simulink model "c960x4096_x14_7_r2013b_frb"  (R2013b)
settings: Solver=ode45  StartTime=0.0  StopTime=40960  RelTol=1e-3
undefined symbols (not defined in the file): sfp
libraries: xbsIndex_r4 x14620, casper_library_misc x61, dspsigops x32, casper_library_multipliers x24, simulink x18, xps_library x18
(part 70 of 79)

== system c960x4096_x14_7_r2013b_frb/vacc/vacc/yy/bit_sel2/bus_expand1 ==
  bus_in : Inport
  reinterpret{1..64} (64 alike) : xbsIndex_r4/Reinterpret  force_arith_type=on  arith_type=Unsigned  force_bin_pt=on  bin_pt=0  block_type=reinterpret
  slice1 : xbsIndex_r4/Slice  nbits=1  boolean_output=off  mode=Upper Bit Location + Width  bit1=-63  base1=MSB of Input  bit0=0  base0=LSB of Input  dbl_ovrd=off  block_type=slice
  slice10 : xbsIndex_r4/Slice  nbits=1  boolean_output=off  mode=Upper Bit Location + Width  bit1=-54  base1=MSB of Input  bit0=0  base0=LSB of Input  dbl_ovrd=off  block_type=slice
  slice11 : xbsIndex_r4/Slice  nbits=1  boolean_output=off  mode=Upper Bit Location + Width  bit1=-53  base1=MSB of Input  bit0=0  base0=LSB of Input  dbl_ovrd=off  block_type=slice
  slice12 : xbsIndex_r4/Slice  nbits=1  boolean_output=off  mode=Upper Bit Location + Width  bit1=-52  base1=MSB of Input  bit0=0  base0=LSB of Input  dbl_ovrd=off  block_type=slice
  slice13 : xbsIndex_r4/Slice  nbits=1  boolean_output=off  mode=Upper Bit Location + Width  bit1=-51  base1=MSB of Input  bit0=0  base0=LSB of Input  dbl_ovrd=off  block_type=slice
  slice14 : xbsIndex_r4/Slice  nbits=1  boolean_output=off  mode=Upper Bit Location + Width  bit1=-50  base1=MSB of Input  bit0=0  base0=LSB of Input  dbl_ovrd=off  block_type=slice
  slice15 : xbsIndex_r4/Slice  nbits=1  boolean_output=off  mode=Upper Bit Location + Width  bit1=-49  base1=MSB of Input  bit0=0  base0=LSB of Input  dbl_ovrd=off  block_type=slice
  slice16 : xbsIndex_r4/Slice  nbits=1  boolean_output=off  mode=Upper Bit Location + Width  bit1=-48  base1=MSB of Input  bit0=0  base0=LSB of Input  dbl_ovrd=off  block_type=slice
  slice17 : xbsIndex_r4/Slice  nbits=1  boolean_output=off  mode=Upper Bit Location + Width  bit1=-47  base1=MSB of Input  bit0=0  base0=LSB of Input  dbl_ovrd=off  block_type=slice
  slice18 : xbsIndex_r4/Slice  nbits=1  boolean_output=off  mode=Upper Bit Location + Width  bit1=-46  base1=MSB of Input  bit0=0  base0=LSB of Input  dbl_ovrd=off  block_type=slice
  slice19 : xbsIndex_r4/Slice  nbits=1  boolean_output=off  mode=Upper Bit Location + Width  bit1=-45  base1=MSB of Input  bit0=0  base0=LSB of Input  dbl_ovrd=off  block_type=slice
  slice2 : xbsIndex_r4/Slice  nbits=1  boolean_output=off  mode=Upper Bit Location + Width  bit1=-62  base1=MSB of Input  bit0=0  base0=LSB of Input  dbl_ovrd=off  block_type=slice
  slice20 : xbsIndex_r4/Slice  nbits=1  boolean_output=off  mode=Upper Bit Location + Width  bit1=-44  base1=MSB of Input  bit0=0  base0=LSB of Input  dbl_ovrd=off  block_type=slice
  slice21 : xbsIndex_r4/Slice  nbits=1  boolean_output=off  mode=Upper Bit Location + Width  bit1=-43  base1=MSB of Input  bit0=0  base0=LSB of Input  dbl_ovrd=off  block_type=slice
  slice22 : xbsIndex_r4/Slice  nbits=1  boolean_output=off  mode=Upper Bit Location + Width  bit1=-42  base1=MSB of Input  bit0=0  base0=LSB of Input  dbl_ovrd=off  block_type=slice
  slice23 : xbsIndex_r4/Slice  nbits=1  boolean_output=off  mode=Upper Bit Location + Width  bit1=-41  base1=MSB of Input  bit0=0  base0=LSB of Input  dbl_ovrd=off  block_type=slice
  slice24 : xbsIndex_r4/Slice  nbits=1  boolean_output=off  mode=Upper Bit Location + Width  bit1=-40  base1=MSB of Input  bit0=0  base0=LSB of Input  dbl_ovrd=off  block_type=slice
  slice25 : xbsIndex_r4/Slice  nbits=1  boolean_output=off  mode=Upper Bit Location + Width  bit1=-39  base1=MSB of Input  bit0=0  base0=LSB of Input  dbl_ovrd=off  block_type=slice
  slice26 : xbsIndex_r4/Slice  nbits=1  boolean_output=off  mode=Upper Bit Location + Width  bit1=-38  base1=MSB of Input  bit0=0  base0=LSB of Input  dbl_ovrd=off  block_type=slice
  slice27 : xbsIndex_r4/Slice  nbits=1  boolean_output=off  mode=Upper Bit Location + Width  bit1=-37  base1=MSB of Input  bit0=0  base0=LSB of Input  dbl_ovrd=off  block_type=slice
  slice28 : xbsIndex_r4/Slice  nbits=1  boolean_output=off  mode=Upper Bit Location + Width  bit1=-36  base1=MSB of Input  bit0=0  base0=LSB of Input  dbl_ovrd=off  block_type=slice
  slice29 : xbsIndex_r4/Slice  nbits=1  boolean_output=off  mode=Upper Bit Location + Width  bit1=-35  base1=MSB of Input  bit0=0  base0=LSB of Input  dbl_ovrd=off  block_type=slice
  slice3 : xbsIndex_r4/Slice  nbits=1  boolean_output=off  mode=Upper Bit Location + Width  bit1=-61  base1=MSB of Input  bit0=0  base0=LSB of Input  dbl_ovrd=off  block_type=slice
  slice30 : xbsIndex_r4/Slice  nbits=1  boolean_output=off  mode=Upper Bit Location + Width  bit1=-34  base1=MSB of Input  bit0=0  base0=LSB of Input  dbl_ovrd=off  block_type=slice
  slice31 : xbsIndex_r4/Slice  nbits=1  boolean_output=off  mode=Upper Bit Location + Width  bit1=-33  base1=MSB of Input  bit0=0  base0=LSB of Input  dbl_ovrd=off  block_type=slice
  slice32 : xbsIndex_r4/Slice  nbits=1  boolean_output=off  mode=Upper Bit Location + Width  bit1=-32  base1=MSB of Input  bit0=0  base0=LSB of Input  dbl_ovrd=off  block_type=slice
  slice33 : xbsIndex_r4/Slice  nbits=1  boolean_output=off  mode=Upper Bit Location + Width  bit1=-31  base1=MSB of Input  bit0=0  base0=LSB of Input  dbl_ovrd=off  block_type=slice
  slice34 : xbsIndex_r4/Slice  nbits=1  boolean_output=off  mode=Upper Bit Location + Width  bit1=-30  base1=MSB of Input  bit0=0  base0=LSB of Input  dbl_ovrd=off  block_type=slice
  slice35 : xbsIndex_r4/Slice  nbits=1  boolean_output=off  mode=Upper Bit Location + Width  bit1=-29  base1=MSB of Input  bit0=0  base0=LSB of Input  dbl_ovrd=off  block_type=slice
  slice36 : xbsIndex_r4/Slice  nbits=1  boolean_output=off  mode=Upper Bit Location + Width  bit1=-28  base1=MSB of Input  bit0=0  base0=LSB of Input  dbl_ovrd=off  block_type=slice
  slice37 : xbsIndex_r4/Slice  nbits=1  boolean_output=off  mode=Upper Bit Location + Width  bit1=-27  base1=MSB of Input  bit0=0  base0=LSB of Input  dbl_ovrd=off  block_type=slice
  slice38 : xbsIndex_r4/Slice  nbits=1  boolean_output=off  mode=Upper Bit Location + Width  bit1=-26  base1=MSB of Input  bit0=0  base0=LSB of Input  dbl_ovrd=off  block_type=slice
  slice39 : xbsIndex_r4/Slice  nbits=1  boolean_output=off  mode=Upper Bit Location + Width  bit1=-25  base1=MSB of Input  bit0=0  base0=LSB of Input  dbl_ovrd=off  block_type=slice
  slice4 : xbsIndex_r4/Slice  nbits=1  boolean_output=off  mode=Upper Bit Location + Width  bit1=-60  base1=MSB of Input  bit0=0  base0=LSB of Input  dbl_ovrd=off  block_type=slice
  slice40 : xbsIndex_r4/Slice  nbits=1  boolean_output=off  mode=Upper Bit Location + Width  bit1=-24  base1=MSB of Input  bit0=0  base0=LSB of Input  dbl_ovrd=off  block_type=slice
  slice41 : xbsIndex_r4/Slice  nbits=1  boolean_output=off  mode=Upper Bit Location + Width  bit1=-23  base1=MSB of Input  bit0=0  base0=LSB of Input  dbl_ovrd=off  block_type=slice
  slice42 : xbsIndex_r4/Slice  nbits=1  boolean_output=off  mode=Upper Bit Location + Width  bit1=-22  base1=MSB of Input  bit0=0  base0=LSB of Input  dbl_ovrd=off  block_type=slice
  slice43 : xbsIndex_r4/Slice  nbits=1  boolean_output=off  mode=Upper Bit Location + Width  bit1=-21  base1=MSB of Input  bit0=0  base0=LSB of Input  dbl_ovrd=off  block_type=slice
  slice44 : xbsIndex_r4/Slice  nbits=1  boolean_output=off  mode=Upper Bit Location + Width  bit1=-20  base1=MSB of Input  bit0=0  base0=LSB of Input  dbl_ovrd=off  block_type=slice
  slice45 : xbsIndex_r4/Slice  nbits=1  boolean_output=off  mode=Upper Bit Location + Width  bit1=-19  base1=MSB of Input  bit0=0  base0=LSB of Input  dbl_ovrd=off  block_type=slice
  slice46 : xbsIndex_r4/Slice  nbits=1  boolean_output=off  mode=Upper Bit Location + Width  bit1=-18  base1=MSB of Input  bit0=0  base0=LSB of Input  dbl_ovrd=off  block_type=slice
  slice47 : xbsIndex_r4/Slice  nbits=1  boolean_output=off  mode=Upper Bit Location + Width  bit1=-17  base1=MSB of Input  bit0=0  base0=LSB of Input  dbl_ovrd=off  block_type=slice
  slice48 : xbsIndex_r4/Slice  nbits=1  boolean_output=off  mode=Upper Bit Location + Width  bit1=-16  base1=MSB of Input  bit0=0  base0=LSB of Input  dbl_ovrd=off  block_type=slice
  slice49 : xbsIndex_r4/Slice  nbits=1  boolean_output=off  mode=Upper Bit Location + Width  bit1=-15  base1=MSB of Input  bit0=0  base0=LSB of Input  dbl_ovrd=off  block_type=slice
  slice5 : xbsIndex_r4/Slice  nbits=1  boolean_output=off  mode=Upper Bit Location + Width  bit1=-59  base1=MSB of Input  bit0=0  base0=LSB of Input  dbl_ovrd=off  block_type=slice
  slice50 : xbsIndex_r4/Slice  nbits=1  boolean_output=off  mode=Upper Bit Location + Width  bit1=-14  base1=MSB of Input  bit0=0  base0=LSB of Input  dbl_ovrd=off  block_type=slice
  slice51 : xbsIndex_r4/Slice  nbits=1  boolean_output=off  mode=Upper Bit Location + Width  bit1=-13  base1=MSB of Input  bit0=0  base0=LSB of Input  dbl_ovrd=off  block_type=slice
  slice52 : xbsIndex_r4/Slice  nbits=1  boolean_output=off  mode=Upper Bit Location + Width  bit1=-12  base1=MSB of Input  bit0=0  base0=LSB of Input  dbl_ovrd=off  block_type=slice
  slice53 : xbsIndex_r4/Slice  nbits=1  boolean_output=off  mode=Upper Bit Location + Width  bit1=-11  base1=MSB of Input  bit0=0  base0=LSB of Input  dbl_ovrd=off  block_type=slice
  slice54 : xbsIndex_r4/Slice  nbits=1  boolean_output=off  mode=Upper Bit Location + Width  bit1=-10  base1=MSB of Input  bit0=0  base0=LSB of Input  dbl_ovrd=off  block_type=slice
  slice55 : xbsIndex_r4/Slice  nbits=1  boolean_output=off  mode=Upper Bit Location + Width  bit1=-9  base1=MSB of Input  bit0=0  base0=LSB of Input  dbl_ovrd=off  block_type=slice
  slice56 : xbsIndex_r4/Slice  nbits=1  boolean_output=off  mode=Upper Bit Location + Width  bit1=-8  base1=MSB of Input  bit0=0  base0=LSB of Input  dbl_ovrd=off  block_type=slice
  slice57 : xbsIndex_r4/Slice  nbits=1  boolean_output=off  mode=Upper Bit Location + Width  bit1=-7  base1=MSB of Input  bit0=0  base0=LSB of Input  dbl_ovrd=off  block_type=slice
  slice58 : xbsIndex_r4/Slice  nbits=1  boolean_output=off  mode=Upper Bit Location + Width  bit1=-6  base1=MSB of Input  bit0=0  base0=LSB of Input  dbl_ovrd=off  block_type=slice
  slice59 : xbsIndex_r4/Slice  nbits=1  boolean_output=off  mode=Upper Bit Location + Width  bit1=-5  base1=MSB of Input  bit0=0  base0=LSB of Input  dbl_ovrd=off  block_type=slice
  slice6 : xbsIndex_r4/Slice  nbits=1  boolean_output=off  mode=Upper Bit Location + Width  bit1=-58  base1=MSB of Input  bit0=0  base0=LSB of Input  dbl_ovrd=off  block_type=slice
  slice60 : xbsIndex_r4/Slice  nbits=1  boolean_output=off  mode=Upper Bit Location + Width  bit1=-4  base1=MSB of Input  bit0=0  base0=LSB of Input  dbl_ovrd=off  block_type=slice
  slice61 : xbsIndex_r4/Slice  nbits=1  boolean_output=off  mode=Upper Bit Location + Width  bit1=-3  base1=MSB of Input  bit0=0  base0=LSB of Input  dbl_ovrd=off  block_type=slice
  slice62 : xbsIndex_r4/Slice  nbits=1  boolean_output=off  mode=Upper Bit Location + Width  bit1=-2  base1=MSB of Input  bit0=0  base0=LSB of Input  dbl_ovrd=off  block_type=slice
  slice63 : xbsIndex_r4/Slice  nbits=1  boolean_output=off  mode=Upper Bit Location + Width  bit1=-1  base1=MSB of Input  bit0=0  base0=LSB of Input  dbl_ovrd=off  block_type=slice
  slice64 : xbsIndex_r4/Slice  nbits=1  boolean_output=off  mode=Upper Bit Location + Width  bit1=0  base1=MSB of Input  bit0=0  base0=LSB of Input  dbl_ovrd=off  block_type=slice
  slice7 : xbsIndex_r4/Slice  nbits=1  boolean_output=off  mode=Upper Bit Location + Width  bit1=-57  base1=MSB of Input  bit0=0  base0=LSB of Input  dbl_ovrd=off  block_type=slice
  slice8 : xbsIndex_r4/Slice  nbits=1  boolean_output=off  mode=Upper Bit Location + Width  bit1=-56  base1=MSB of Input  bit0=0  base0=LSB of Input  dbl_ovrd=off  block_type=slice
  slice9 : xbsIndex_r4/Slice  nbits=1  boolean_output=off  mode=Upper Bit Location + Width  bit1=-55  base1=MSB of Input  bit0=0  base0=LSB of Input  dbl_ovrd=off  block_type=slice
  msb_out64 : Outport
  out63 : Outport  Port=2
  out62 : Outport  Port=3
  out61 : Outport  Port=4
  out60 : Outport  Port=5
  out59 : Outport  Port=6
  out58 : Outport  Port=7
  out57 : Outport  Port=8
  out56 : Outport  Port=9
  out55 : Outport  Port=10
  out54 : Outport  Port=11
  out53 : Outport  Port=12
  out52 : Outport  Port=13
  out51 : Outport  Port=14
  out50 : Outport  Port=15
  out49 : Outport  Port=16
  out48 : Outport  Port=17
  out47 : Outport  Port=18
  out46 : Outport  Port=19
  out45 : Outport  Port=20
  out44 : Outport  Port=21
  out43 : Outport  Port=22
  out42 : Outport  Port=23
  out41 : Outport  Port=24
  out40 : Outport  Port=25
  out39 : Outport  Port=26
  out38 : Outport  Port=27
  out37 : Outport  Port=28
  out36 : Outport  Port=29
  out35 : Outport  Port=30
  out34 : Outport  Port=31
  out33 : Outport  Port=32
  out32 : Outport  Port=33
  out31 : Outport  Port=34
  out30 : Outport  Port=35
  out29 : Outport  Port=36
  out28 : Outport  Port=37
  out27 : Outport  Port=38
  out26 : Outport  Port=39
  out25 : Outport  Port=40
  out24 : Outport  Port=41
  out23 : Outport  Port=42
  out22 : Outport  Port=43
  out21 : Outport  Port=44
  out20 : Outport  Port=45
  out19 : Outport  Port=46
  out18 : Outport  Port=47
  out17 : Outport  Port=48
  out16 : Outport  Port=49
  out15 : Outport  Port=50
  out14 : Outport  Port=51
  out13 : Outport  Port=52
  out12 : Outport  Port=53
  out11 : Outport  Port=54
  out10 : Outport  Port=55
  out9 : Outport  Port=56
  out8 : Outport  Port=57
  out7 : Outport  Port=58
  out6 : Outport  Port=59
  out5 : Outport  Port=60
  out4 : Outport  Port=61
  out3 : Outport  Port=62
  out2 : Outport  Port=63
  lsb_out1 : Outport  Port=64
  wires:
  bus_in/1 -> slice64/1, slice63/1, slice62/1, slice61/1, slice60/1, slice59/1, slice58/1, slice57/1, slice56/1, slice55/1, slice54/1, slice53/1, slice52/1, slice51/1, slice50/1, slice49/1, slice48/1, slice47/1, slice46/1, slice45/1, slice44/1, slice43/1, slice42/1, slice41/1, slice40/1, slice39/1, slice38/1, slice37/1, slice36/1, slice35/1, slice34/1, slice33/1, slice32/1, slice31/1, slice30/1, slice29/1, slice28/1, slice27/1, slice26/1, slice25/1, slice24/1, slice23/1, slice22/1, slice21/1, slice20/1, slice19/1, slice18/1, slice17/1, slice16/1, slice15/1, slice14/1, slice13/1, slice12/1, slice11/1, slice10/1, slice9/1, slice8/1, slice7/1, slice6/1, slice5/1, slice4/1, slice3/1, slice2/1, slice1/1
  slice64/1 -> reinterpret64/1
  reinterpret64/1 -> msb_out64/1
  slice63/1 -> reinterpret63/1
  reinterpret63/1 -> out63/1
  slice62/1 -> reinterpret62/1
  reinterpret62/1 -> out62/1
  slice61/1 -> reinterpret61/1
  reinterpret61/1 -> out61/1
  slice60/1 -> reinterpret60/1
  reinterpret60/1 -> out60/1
  slice59/1 -> reinterpret59/1
  reinterpret59/1 -> out59/1
  slice58/1 -> reinterpret58/1
  reinterpret58/1 -> out58/1
  slice57/1 -> reinterpret57/1
  reinterpret57/1 -> out57/1
  slice56/1 -> reinterpret56/1
  reinterpret56/1 -> out56/1
  slice55/1 -> reinterpret55/1
  reinterpret55/1 -> out55/1
  slice54/1 -> reinterpret54/1
  reinterpret54/1 -> out54/1
  slice53/1 -> reinterpret53/1
  reinterpret53/1 -> out53/1
  slice52/1 -> reinterpret52/1
  reinterpret52/1 -> out52/1
  slice51/1 -> reinterpret51/1
  reinterpret51/1 -> out51/1
  slice50/1 -> reinterpret50/1
  reinterpret50/1 -> out50/1
  slice49/1 -> reinterpret49/1
  reinterpret49/1 -> out49/1
  slice48/1 -> reinterpret48/1
  reinterpret48/1 -> out48/1
  slice47/1 -> reinterpret47/1
  reinterpret47/1 -> out47/1
  slice46/1 -> reinterpret46/1
  reinterpret46/1 -> out46/1
  slice45/1 -> reinterpret45/1
  reinterpret45/1 -> out45/1
  slice44/1 -> reinterpret44/1
  reinterpret44/1 -> out44/1
  slice43/1 -> reinterpret43/1
  reinterpret43/1 -> out43/1
  slice42/1 -> reinterpret42/1
  reinterpret42/1 -> out42/1
  slice41/1 -> reinterpret41/1
  reinterpret41/1 -> out41/1
  slice40/1 -> reinterpret40/1
  reinterpret40/1 -> out40/1
  slice39/1 -> reinterpret39/1
  reinterpret39/1 -> out39/1
  slice38/1 -> reinterpret38/1
  reinterpret38/1 -> out38/1
  slice37/1 -> reinterpret37/1
  reinterpret37/1 -> out37/1
  slice36/1 -> reinterpret36/1
  reinterpret36/1 -> out36/1
  slice35/1 -> reinterpret35/1
  reinterpret35/1 -> out35/1
  slice34/1 -> reinterpret34/1
  reinterpret34/1 -> out34/1
  slice33/1 -> reinterpret33/1
  reinterpret33/1 -> out33/1
  slice32/1 -> reinterpret32/1
  reinterpret32/1 -> out32/1
  slice31/1 -> reinterpret31/1
  reinterpret31/1 -> out31/1
  slice30/1 -> reinterpret30/1
  reinterpret30/1 -> out30/1
  slice29/1 -> reinterpret29/1
  reinterpret29/1 -> out29/1
  slice28/1 -> reinterpret28/1
  reinterpret28/1 -> out28/1
  slice27/1 -> reinterpret27/1
  reinterpret27/1 -> out27/1
  slice26/1 -> reinterpret26/1
  reinterpret26/1 -> out26/1
  slice25/1 -> reinterpret25/1
  reinterpret25/1 -> out25/1
  slice24/1 -> reinterpret24/1
  reinterpret24/1 -> out24/1
  slice23/1 -> reinterpret23/1
  reinterpret23/1 -> out23/1
  slice22/1 -> reinterpret22/1
  reinterpret22/1 -> out22/1
  slice21/1 -> reinterpret21/1
  reinterpret21/1 -> out21/1
  slice20/1 -> reinterpret20/1
  reinterpret20/1 -> out20/1
  slice19/1 -> reinterpret19/1
  reinterpret19/1 -> out19/1
  slice18/1 -> reinterpret18/1
  reinterpret18/1 -> out18/1
  slice17/1 -> reinterpret17/1
  reinterpret17/1 -> out17/1
  slice16/1 -> reinterpret16/1
  reinterpret16/1 -> out16/1
  slice15/1 -> reinterpret15/1
  reinterpret15/1 -> out15/1
  slice14/1 -> reinterpret14/1
  reinterpret14/1 -> out14/1
  slice13/1 -> reinterpret13/1
  reinterpret13/1 -> out13/1
  slice12/1 -> reinterpret12/1
  reinterpret12/1 -> out12/1
  slice11/1 -> reinterpret11/1
  reinterpret11/1 -> out11/1
  slice10/1 -> reinterpret10/1
  reinterpret10/1 -> out10/1
  slice9/1 -> reinterpret9/1
  reinterpret9/1 -> out9/1
  slice8/1 -> reinterpret8/1
  reinterpret8/1 -> out8/1
  slice7/1 -> reinterpret7/1
  reinterpret7/1 -> out7/1
  slice6/1 -> reinterpret6/1
  reinterpret6/1 -> out6/1
  slice5/1 -> reinterpret5/1
  reinterpret5/1 -> out5/1
  slice4/1 -> reinterpret4/1
  reinterpret4/1 -> out4/1
  slice3/1 -> reinterpret3/1
  reinterpret3/1 -> out3/1
  slice2/1 -> reinterpret2/1
  reinterpret2/1 -> out2/1
  slice1/1 -> reinterpret1/1
  reinterpret1/1 -> lsb_out1/1

== system c960x4096_x14_7_r2013b_frb/vacc/vacc/yy/bit_sel3/barrel_switcher ==
  sel : Inport
  sync_in : Inport  Port=2
  In1 : Inport  Port=3
  In2 : Inport  Port=4
  In3 : Inport  Port=5
  In4 : Inport  Port=6
  In5 : Inport  Port=7
  In6 : Inport  Port=8
  In7 : Inport  Port=9
  In8 : Inport  Port=10
  In9 : Inport  Port=11
  In10 : Inport  Port=12
  In11 : Inport  Port=13
  In12 : Inport  Port=14
  In13 : Inport  Port=15
  In14 : Inport  Port=16
  In15 : Inport  Port=17
  In16 : Inport  Port=18
  In17 : Inport  Port=19
  In18 : Inport  Port=20
  In19 : Inport  Port=21
  In20 : Inport  Port=22
  In21 : Inport  Port=23
  In22 : Inport  Port=24
  In23 : Inport  Port=25
  In24 : Inport  Port=26
  In25 : Inport  Port=27
  In26 : Inport  Port=28
  In27 : Inport  Port=29
  In28 : Inport  Port=30
  In29 : Inport  Port=31
  In30 : Inport  Port=32
  In31 : Inport  Port=33
  In32 : Inport  Port=34
  In33 : Inport  Port=35
  In34 : Inport  Port=36
  In35 : Inport  Port=37
  In36 : Inport  Port=38
  In37 : Inport  Port=39
  In38 : Inport  Port=40
  In39 : Inport  Port=41
  In40 : Inport  Port=42
  In41 : Inport  Port=43
  In42 : Inport  Port=44
  In43 : Inport  Port=45
  In44 : Inport  Port=46
  In45 : Inport  Port=47
  In46 : Inport  Port=48
  In47 : Inport  Port=49
  In48 : Inport  Port=50
  In49 : Inport  Port=51
  In50 : Inport  Port=52
  In51 : Inport  Port=53
  In52 : Inport  Port=54
  In53 : Inport  Port=55
  In54 : Inport  Port=56
  In55 : Inport  Port=57
  In56 : Inport  Port=58
  In57 : Inport  Port=59
  In58 : Inport  Port=60
  In59 : Inport  Port=61
  In60 : Inport  Port=62
  In61 : Inport  Port=63
  In62 : Inport  Port=64
  In63 : Inport  Port=65
  In64 : Inport  Port=66
  Delay{1..5} (5 alike) : xbsIndex_r4/Delay  rst=off  infoeditControl=Selection of Reset will increase slice count due to use of real FFs and instead of SRLs  en=off  latency=1  dbl_ovrd=off  reg_retiming=on  block_type=delay
  Delay_sync : xbsIndex_r4/Delay  rst=off  infoeditControl=Selection of Reset will increase slice count due to use of real FFs and instead of SRLs  en=off  latency=6  dbl_ovrd=off  reg_retiming=on  block_type=delay
  Mux{11..16,21..26,31..36,41..46,51..56,61..66,71..76,81..86,91..96,101..106,111..116,121..126,131..136,141..146,151..156,161..166,171..176,181..186,191..196,201..206,211..216,221..226,231..236,241..246,251..256,261..266,271..276,281..286,291..296,301..306,311..316,321..326,331..336,341..346,351..356,361..366,371..376,381..386,391..396,401..406,411..416,421..426,431..436,441..446,451..456,461..466,471..476,481..486,491..496,501..506,511..516,521..526,531..536,541..546,551..556,561..566,571..576,581..586,591..596,601..606,611..616,621..626,631..636,641..646} (384 alike) : xbsIndex_r4/Mux  inputs=2  en=off  latency=1  precision=Full  arith_type=Unsigned  n_bits=16  bin_pt=14  quantization=Truncate  overflow=Wrap  dbl_ovrd=off  block_type=mux
  Slice1 : xbsIndex_r4/Slice  nbits=1  boolean_output=off  mode=Upper Bit Location + Width  bit1=-0  base1=MSB of Input  bit0=0  base0=LSB of Input  dbl_ovrd=off  block_type=slice
  Slice2 : xbsIndex_r4/Slice  nbits=1  boolean_output=off  mode=Upper Bit Location + Width  bit1=-1  base1=MSB of Input  bit0=0  base0=LSB of Input  dbl_ovrd=off  block_type=slice
  Slice3 : xbsIndex_r4/Slice  nbits=1  boolean_output=off  mode=Upper Bit Location + Width  bit1=-2  base1=MSB of Input  bit0=0  base0=LSB of Input  dbl_ovrd=off  block_type=slice
  Slice4 : xbsIndex_r4/Slice  nbits=1  boolean_output=off  mode=Upper Bit Location + Width  bit1=-3  base1=MSB of Input  bit0=0  base0=LSB of Input  dbl_ovrd=off  block_type=slice
  Slice5 : xbsIndex_r4/Slice  nbits=1  boolean_output=off  mode=Upper Bit Location + Width  bit1=-4  base1=MSB of Input  bit0=0  base0=LSB of Input  dbl_ovrd=off  block_type=slice
  Slice6 : xbsIndex_r4/Slice  nbits=1  boolean_output=off  mode=Upper Bit Location + Width  bit1=-5  base1=MSB of Input  bit0=0  base0=LSB of Input  dbl_ovrd=off  block_type=slice
  sync_out : Outport
  Out1 : Outport  Port=2
  Out2 : Outport  Port=3
  Out3 : Outport  Port=4
  Out4 : Outport  Port=5
  Out5 : Outport  Port=6
  Out6 : Outport  Port=7
  Out7 : Outport  Port=8
  Out8 : Outport  Port=9
  Out9 : Outport  Port=10
  Out10 : Outport  Port=11
  Out11 : Outport  Port=12
  Out12 : Outport  Port=13
  Out13 : Outport  Port=14
  Out14 : Outport  Port=15
  Out15 : Outport  Port=16
  Out16 : Outport  Port=17
  Out17 : Outport  Port=18
  Out18 : Outport  Port=19
  Out19 : Outport  Port=20
  Out20 : Outport  Port=21
  Out21 : Outport  Port=22
  Out22 : Outport  Port=23
  Out23 : Outport  Port=24
  Out24 : Outport  Port=25
  Out25 : Outport  Port=26
  Out26 : Outport  Port=27
  Out27 : Outport  Port=28
  Out28 : Outport  Port=29
  Out29 : Outport  Port=30
  Out30 : Outport  Port=31
  Out31 : Outport  Port=32
  Out32 : Outport  Port=33
  Out33 : Outport  Port=34
  Out34 : Outport  Port=35
  Out35 : Outport  Port=36
  Out36 : Outport  Port=37
  Out37 : Outport  Port=38
  Out38 : Outport  Port=39
  Out39 : Outport  Port=40
  Out40 : Outport  Port=41
  Out41 : Outport  Port=42
  Out42 : Outport  Port=43
  Out43 : Outport  Port=44
  Out44 : Outport  Port=45
  Out45 : Outport  Port=46
  Out46 : Outport  Port=47
  Out47 : Outport  Port=48
  Out48 : Outport  Port=49
  Out49 : Outport  Port=50
  Out50 : Outport  Port=51
  Out51 : Outport  Port=52
  Out52 : Outport  Port=53
  Out53 : Outport  Port=54
  Out54 : Outport  Port=55
  Out55 : Outport  Port=56
  Out56 : Outport  Port=57
  Out57 : Outport  Port=58
  Out58 : Outport  Port=59
  Out59 : Outport  Port=60
  Out60 : Outport  Port=61
  Out61 : Outport  Port=62
  Out62 : Outport  Port=63
  Out63 : Outport  Port=64
  Out64 : Outport  Port=65
  wires:
  sync_in/1 -> Delay_sync/1
  Delay_sync/1 -> sync_out/1
  sel/1 -> Slice1/1, Delay1/1
  Delay1/1 -> Delay2/1, Slice2/1
  Delay2/1 -> Delay3/1, Slice3/1
  Delay3/1 -> Delay4/1, Slice4/1
  Delay4/1 -> Delay5/1, Slice5/1
  Delay5/1 -> Slice6/1
  Slice1/1 -> Mux11/1, Mux21/1, Mux31/1, Mux41/1, Mux51/1, Mux61/1, Mux71/1, Mux81/1, Mux91/1, Mux101/1, Mux111/1, Mux121/1, Mux131/1, Mux141/1, Mux151/1, Mux161/1, Mux171/1, Mux181/1, Mux191/1, Mux201/1, Mux211/1, Mux221/1, Mux231/1, Mux241/1, Mux251/1, Mux261/1, Mux271/1, Mux281/1, Mux291/1, Mux301/1, Mux311/1, Mux321/1, Mux331/1, Mux341/1, Mux351/1, Mux361/1, Mux371/1, Mux381/1, Mux391/1, Mux401/1, Mux411/1, Mux421/1, Mux431/1, Mux441/1, Mux451/1, Mux461/1, Mux471/1, Mux481/1, Mux491/1, Mux501/1, Mux511/1, Mux521/1, Mux531/1, Mux541/1, Mux551/1, Mux561/1, Mux571/1, Mux581/1, Mux591/1, Mux601/1, Mux611/1, Mux621/1, Mux631/1, Mux641/1
  Slice2/1 -> Mux12/1, Mux22/1, Mux32/1, Mux42/1, Mux52/1, Mux62/1, Mux72/1, Mux82/1, Mux92/1, Mux102/1, Mux112/1, Mux122/1, Mux132/1, Mux142/1, Mux152/1, Mux162/1, Mux172/1, Mux182/1, Mux192/1, Mux202/1, Mux212/1, Mux222/1, Mux232/1, Mux242/1, Mux252/1, Mux262/1, Mux272/1, Mux282/1, Mux292/1, Mux302/1, Mux312/1, Mux322/1, Mux332/1, Mux342/1, Mux352/1, Mux362/1, Mux372/1, Mux382/1, Mux392/1, Mux402/1, Mux412/1, Mux422/1, Mux432/1, Mux442/1, Mux452/1, Mux462/1, Mux472/1, Mux482/1, Mux492/1, Mux502/1, Mux512/1, Mux522/1, Mux532/1, Mux542/1, Mux552/1, Mux562/1, Mux572/1, Mux582/1, Mux592/1, Mux602/1, Mux612/1, Mux622/1, Mux632/1, Mux642/1
  Slice3/1 -> Mux13/1, Mux23/1, Mux33/1, Mux43/1, Mux53/1, Mux63/1, Mux73/1, Mux83/1, Mux93/1, Mux103/1, Mux113/1, Mux123/1, Mux133/1, Mux143/1, Mux153/1, Mux163/1, Mux173/1, Mux183/1, Mux193/1, Mux203/1, Mux213/1, Mux223/1, Mux233/1, Mux243/1, Mux253/1, Mux263/1, Mux273/1, Mux283/1, Mux293/1, Mux303/1, Mux313/1, Mux323/1, Mux333/1, Mux343/1, Mux353/1, Mux363/1, Mux373/1, Mux383/1, Mux393/1, Mux403/1, Mux413/1, Mux423/1, Mux433/1, Mux443/1, Mux453/1, Mux463/1, Mux473/1, Mux483/1, Mux493/1, Mux503/1, Mux513/1, Mux523/1, Mux533/1, Mux543/1, Mux553/1, Mux563/1, Mux573/1, Mux583/1, Mux593/1, Mux603/1, Mux613/1, Mux623/1, Mux633/1, Mux643/1
  Slice4/1 -> Mux14/1, Mux24/1, Mux34/1, Mux44/1, Mux54/1, Mux64/1, Mux74/1, Mux84/1, Mux94/1, Mux104/1, Mux114/1, Mux124/1, Mux134/1, Mux144/1, Mux154/1, Mux164/1, Mux174/1, Mux184/1, Mux194/1, Mux204/1, Mux214/1, Mux224/1, Mux234/1, Mux244/1, Mux254/1, Mux264/1, Mux274/1, Mux284/1, Mux294/1, Mux304/1, Mux314/1, Mux324/1, Mux334/1, Mux344/1, Mux354/1, Mux364/1, Mux374/1, Mux384/1, Mux394/1, Mux404/1, Mux414/1, Mux424/1, Mux434/1, Mux444/1, Mux454/1, Mux464/1, Mux474/1, Mux484/1, Mux494/1, Mux504/1, Mux514/1, Mux524/1, Mux534/1, Mux544/1, Mux554/1, Mux564/1, Mux574/1, Mux584/1, Mux594/1, Mux604/1, Mux614/1, Mux624/1, Mux634/1, Mux644/1
  Slice5/1 -> Mux15/1, Mux25/1, Mux35/1, Mux45/1, Mux55/1, Mux65/1, Mux75/1, Mux85/1, Mux95/1, Mux105/1, Mux115/1, Mux125/1, Mux135/1, Mux145/1, Mux155/1, Mux165/1, Mux175/1, Mux185/1, Mux195/1, Mux205/1, Mux215/1, Mux225/1, Mux235/1, Mux245/1, Mux255/1, Mux265/1, Mux275/1, Mux285/1, Mux295/1, Mux305/1, Mux315/1, Mux325/1, Mux335/1, Mux345/1, Mux355/1, Mux365/1, Mux375/1, Mux385/1, Mux395/1, Mux405/1, Mux415/1, Mux425/1, Mux435/1, Mux445/1, Mux455/1, Mux465/1, Mux475/1, Mux485/1, Mux495/1, Mux505/1, Mux515/1, Mux525/1, Mux535/1, Mux545/1, Mux555/1, Mux565/1, Mux575/1, Mux585/1, Mux595/1, Mux605/1, Mux615/1, Mux625/1, Mux635/1, Mux645/1
  Slice6/1 -> Mux16/1, Mux26/1, Mux36/1, Mux46/1, Mux56/1, Mux66/1, Mux76/1, Mux86/1, Mux96/1, Mux106/1, Mux116/1, Mux126/1, Mux136/1, Mux146/1, Mux156/1, Mux166/1, Mux176/1, Mux186/1, Mux196/1, Mux206/1, Mux216/1, Mux226/1, Mux236/1, Mux246/1, Mux256/1, Mux266/1, Mux276/1, Mux286/1, Mux296/1, Mux306/1, Mux316/1, Mux326/1, Mux336/1, Mux346/1, Mux356/1, Mux366/1, Mux376/1, Mux386/1, Mux396/1, Mux406/1, Mux416/1, Mux426/1, Mux436/1, Mux446/1, Mux456/1, Mux466/1, Mux476/1, Mux486/1, Mux496/1, Mux506/1, Mux516/1, Mux526/1, Mux536/1, Mux546/1, Mux556/1, Mux566/1, Mux576/1, Mux586/1, Mux596/1, Mux606/1, Mux616/1, Mux626/1, Mux636/1, Mux646/1
  In1/1 -> Mux11/2, Mux331/3
  Mux16/1 -> Out1/1
  In2/1 -> Mux21/2, Mux341/3
  Mux26/1 -> Out2/1
  In3/1 -> Mux31/2, Mux351/3
  Mux36/1 -> Out3/1
  In4/1 -> Mux41/2, Mux361/3
  Mux46/1 -> Out4/1
  In5/1 -> Mux51/2, Mux371/3
  Mux56/1 -> Out5/1
  In6/1 -> Mux61/2, Mux381/3
  Mux66/1 -> Out6/1
  In7/1 -> Mux71/2, Mux391/3
  Mux76/1 -> Out7/1
  In8/1 -> Mux81/2, Mux401/3
  Mux86/1 -> Out8/1
  In9/1 -> Mux91/2, Mux411/3
  Mux96/1 -> Out9/1
  In10/1 -> Mux101/2, Mux421/3
  Mux106/1 -> Out10/1
  In11/1 -> Mux111/2, Mux431/3
  Mux116/1 -> Out11/1
  In12/1 -> Mux121/2, Mux441/3
  Mux126/1 -> Out12/1
  In13/1 -> Mux131/2, Mux451/3
  Mux136/1 -> Out13/1
  In14/1 -> Mux141/2, Mux461/3
  Mux146/1 -> Out14/1
  In15/1 -> Mux151/2, Mux471/3
  Mux156/1 -> Out15/1
  In16/1 -> Mux161/2, Mux481/3
  Mux166/1 -> Out16/1
  In17/1 -> Mux171/2, Mux491/3
  Mux176/1 -> Out17/1
  In18/1 -> Mux181/2, Mux501/3
  Mux186/1 -> Out18/1
  In19/1 -> Mux191/2, Mux511/3
  Mux196/1 -> Out19/1
  In20/1 -> Mux201/2, Mux521/3
  Mux206/1 -> Out20/1
  In21/1 -> Mux211/2, Mux531/3
  Mux216/1 -> Out21/1
  In22/1 -> Mux221/2, Mux541/3
  Mux226/1 -> Out22/1
  In23/1 -> Mux231/2, Mux551/3
  Mux236/1 -> Out23/1
  In24/1 -> Mux241/2, Mux561/3
  Mux246/1 -> Out24/1
  In25/1 -> Mux251/2, Mux571/3
  Mux256/1 -> Out25/1
  In26/1 -> Mux261/2, Mux581/3
  Mux266/1 -> Out26/1
  In27/1 -> Mux271/2, Mux591/3
  Mux276/1 -> Out27/1
  In28/1 -> Mux281/2, Mux601/3
  Mux286/1 -> Out28/1
  In29/1 -> Mux291/2, Mux611/3
  Mux296/1 -> Out29/1
  In30/1 -> Mux301/2, Mux621/3
  Mux306/1 -> Out30/1
  In31/1 -> Mux311/2, Mux631/3
  Mux316/1 -> Out31/1
  In32/1 -> Mux321/2, Mux641/3
  Mux326/1 -> Out32/1
  In33/1 -> Mux331/2, Mux11/3
  Mux336/1 -> Out33/1
  In34/1 -> Mux341/2, Mux21/3
  Mux346/1 -> Out34/1
  In35/1 -> Mux351/2, Mux31/3
  Mux356/1 -> Out35/1
  In36/1 -> Mux361/2, Mux41/3
  Mux366/1 -> Out36/1
  In37/1 -> Mux371/2, Mux51/3
  Mux376/1 -> Out37/1
  In38/1 -> Mux381/2, Mux61/3
  Mux386/1 -> Out38/1
  In39/1 -> Mux391/2, Mux71/3
  Mux396/1 -> Out39/1
  In40/1 -> Mux401/2, Mux81/3
  Mux406/1 -> Out40/1
  In41/1 -> Mux411/2, Mux91/3
  Mux416/1 -> Out41/1
  In42/1 -> Mux421/2, Mux101/3
  Mux426/1 -> Out42/1
  In43/1 -> Mux431/2, Mux111/3
  Mux436/1 -> Out43/1
  In44/1 -> Mux441/2, Mux121/3
  Mux446/1 -> Out44/1
  In45/1 -> Mux451/2, Mux131/3
  Mux456/1 -> Out45/1
  In46/1 -> Mux461/2, Mux141/3
  Mux466/1 -> Out46/1
  In47/1 -> Mux471/2, Mux151/3
  Mux476/1 -> Out47/1
  In48/1 -> Mux481/2, Mux161/3
  Mux486/1 -> Out48/1
  In49/1 -> Mux491/2, Mux171/3
  Mux496/1 -> Out49/1
  In50/1 -> Mux501/2, Mux181/3
  Mux506/1 -> Out50/1
  In51/1 -> Mux511/2, Mux191/3
  Mux516/1 -> Out51/1
  In52/1 -> Mux521/2, Mux201/3
  Mux526/1 -> Out52/1
  In53/1 -> Mux531/2, Mux211/3
  Mux536/1 -> Out53/1
  In54/1 -> Mux541/2, Mux221/3
  Mux546/1 -> Out54/1
  In55/1 -> Mux551/2, Mux231/3
  Mux556/1 -> Out55/1
  In56/1 -> Mux561/2, Mux241/3
  Mux566/1 -> Out56/1
  In57/1 -> Mux571/2, Mux251/3
  Mux576/1 -> Out57/1
  In58/1 -> Mux581/2, Mux261/3
  Mux586/1 -> Out58/1
  In59/1 -> Mux591/2, Mux271/3
  Mux596/1 -> Out59/1
  In60/1 -> Mux601/2, Mux281/3
  Mux606/1 -> Out60/1
  In61/1 -> Mux611/2, Mux291/3
  Mux616/1 -> Out61/1
  In62/1 -> Mux621/2, Mux301/3
  Mux626/1 -> Out62/1
  In63/1 -> Mux631/2, Mux311/3
  Mux636/1 -> Out63/1
  In64/1 -> Mux641/2, Mux321/3
  Mux646/1 -> Out64/1
  Mux11/1 -> Mux12/2, Mux492/3
  Mux12/1 -> Mux13/2, Mux573/3
  Mux13/1 -> Mux14/2, Mux614/3
  Mux14/1 -> Mux15/2, Mux635/3
  Mux15/1 -> Mux16/2, Mux646/3
  Mux21/1 -> Mux22/2, Mux502/3
  Mux22/1 -> Mux23/2, Mux583/3
  Mux23/1 -> Mux24/2, Mux624/3
  Mux24/1 -> Mux25/2, Mux645/3
  Mux25/1 -> Mux26/2, Mux16/3
  Mux31/1 -> Mux32/2, Mux512/3
  Mux32/1 -> Mux33/2, Mux593/3
  Mux33/1 -> Mux34/2, Mux634/3
  Mux34/1 -> Mux35/2, Mux15/3
  Mux35/1 -> Mux36/2, Mux26/3
  Mux41/1 -> Mux42/2, Mux522/3
  Mux42/1 -> Mux43/2, Mux603/3
  Mux43/1 -> Mux44/2, Mux644/3
  Mux44/1 -> Mux45/2, Mux25/3
  Mux45/1 -> Mux46/2, Mux36/3
  Mux51/1 -> Mux52/2, Mux532/3
  Mux52/1 -> Mux53/2, Mux613/3
  Mux53/1 -> Mux54/2, Mux14/3
  Mux54/1 -> Mux55/2, Mux35/3
  Mux55/1 -> Mux56/2, Mux46/3
  Mux61/1 -> Mux62/2, Mux542/3
  Mux62/1 -> Mux63/2, Mux623/3
  Mux63/1 -> Mux64/2, Mux24/3
  Mux64/1 -> Mux65/2, Mux45/3
  Mux65/1 -> Mux66/2, Mux56/3
  Mux71/1 -> Mux72/2, Mux552/3
  Mux72/1 -> Mux73/2, Mux633/3
  Mux73/1 -> Mux74/2, Mux34/3
  Mux74/1 -> Mux75/2, Mux55/3
  Mux75/1 -> Mux76/2, Mux66/3
  Mux81/1 -> Mux82/2, Mux562/3
  Mux82/1 -> Mux83/2, Mux643/3
  Mux83/1 -> Mux84/2, Mux44/3
  Mux84/1 -> Mux85/2, Mux65/3
  Mux85/1 -> Mux86/2, Mux76/3
  Mux91/1 -> Mux92/2, Mux572/3
  Mux92/1 -> Mux93/2, Mux13/3
  Mux93/1 -> Mux94/2, Mux54/3
  Mux94/1 -> Mux95/2, Mux75/3
  Mux95/1 -> Mux96/2, Mux86/3
  Mux101/1 -> Mux102/2, Mux582/3
  Mux102/1 -> Mux103/2, Mux23/3
  Mux103/1 -> Mux104/2, Mux64/3
  Mux104/1 -> Mux105/2, Mux85/3
  Mux105/1 -> Mux106/2, Mux96/3
  Mux111/1 -> Mux112/2, Mux592/3
  Mux112/1 -> Mux113/2, Mux33/3
  Mux113/1 -> Mux114/2, Mux74/3
  Mux114/1 -> Mux115/2, Mux95/3
  Mux115/1 -> Mux116/2, Mux106/3
  Mux121/1 -> Mux122/2, Mux602/3
  Mux122/1 -> Mux123/2, Mux43/3
  Mux123/1 -> Mux124/2, Mux84/3
  Mux124/1 -> Mux125/2, Mux105/3
  Mux125/1 -> Mux126/2, Mux116/3
  Mux131/1 -> Mux132/2, Mux612/3
  Mux132/1 -> Mux133/2, Mux53/3
  Mux133/1 -> Mux134/2, Mux94/3
  Mux134/1 -> Mux135/2, Mux115/3
  Mux135/1 -> Mux136/2, Mux126/3
  Mux141/1 -> Mux142/2, Mux622/3
  Mux142/1 -> Mux143/2, Mux63/3
  Mux143/1 -> Mux144/2, Mux104/3
  Mux144/1 -> Mux145/2, Mux125/3
  Mux145/1 -> Mux146/2, Mux136/3
  Mux151/1 -> Mux152/2, Mux632/3
  Mux152/1 -> Mux153/2, Mux73/3
  Mux153/1 -> Mux154/2, Mux114/3
  Mux154/1 -> Mux155/2, Mux135/3
  Mux155/1 -> Mux156/2, Mux146/3
  Mux161/1 -> Mux162/2, Mux642/3
  Mux162/1 -> Mux163/2, Mux83/3
  Mux163/1 -> Mux164/2, Mux124/3
  Mux164/1 -> Mux165/2, Mux145/3
  Mux165/1 -> Mux166/2, Mux156/3
  Mux171/1 -> Mux172/2, Mux12/3
  Mux172/1 -> Mux173/2, Mux93/3
  Mux173/1 -> Mux174/2, Mux134/3
  Mux174/1 -> Mux175/2, Mux155/3
  Mux175/1 -> Mux176/2, Mux166/3
  Mux181/1 -> Mux182/2, Mux22/3
  Mux182/1 -> Mux183/2, Mux103/3
  Mux183/1 -> Mux184/2, Mux144/3
  Mux184/1 -> Mux185/2, Mux165/3
  Mux185/1 -> Mux186/2, Mux176/3
  Mux191/1 -> Mux192/2, Mux32/3
  Mux192/1 -> Mux193/2, Mux113/3
  Mux193/1 -> Mux194/2, Mux154/3
  Mux194/1 -> Mux195/2, Mux175/3
  Mux195/1 -> Mux196/2, Mux186/3
  Mux201/1 -> Mux202/2, Mux42/3
  Mux202/1 -> Mux203/2, Mux123/3
  Mux203/1 -> Mux204/2, Mux164/3
  Mux204/1 -> Mux205/2, Mux185/3
  Mux205/1 -> Mux206/2, Mux196/3
  Mux211/1 -> Mux212/2, Mux52/3
  Mux212/1 -> Mux213/2, Mux133/3
  Mux213/1 -> Mux214/2, Mux174/3
  Mux214/1 -> Mux215/2, Mux195/3
  Mux215/1 -> Mux216/2, Mux206/3
  Mux221/1 -> Mux222/2, Mux62/3
  Mux222/1 -> Mux223/2, Mux143/3
  Mux223/1 -> Mux224/2, Mux184/3
  Mux224/1 -> Mux225/2, Mux205/3
  Mux225/1 -> Mux226/2, Mux216/3
  Mux231/1 -> Mux232/2, Mux72/3
  Mux232/1 -> Mux233/2, Mux153/3
  Mux233/1 -> Mux234/2, Mux194/3
  Mux234/1 -> Mux235/2, Mux215/3
  Mux235/1 -> Mux236/2, Mux226/3
  Mux241/1 -> Mux242/2, Mux82/3
  Mux242/1 -> Mux243/2, Mux163/3
  Mux243/1 -> Mux244/2, Mux204/3
  Mux244/1 -> Mux245/2, Mux225/3
  Mux245/1 -> Mux246/2, Mux236/3
  Mux251/1 -> Mux252/2, Mux92/3
  Mux252/1 -> Mux253/2, Mux173/3
  Mux253/1 -> Mux254/2, Mux214/3
  Mux254/1 -> Mux255/2, Mux235/3
  Mux255/1 -> Mux256/2, Mux246/3
  Mux261/1 -> Mux262/2, Mux102/3
  Mux262/1 -> Mux263/2, Mux183/3
  Mux263/1 -> Mux264/2, Mux224/3
  Mux264/1 -> Mux265/2, Mux245/3
  Mux265/1 -> Mux266/2, Mux256/3
  Mux271/1 -> Mux272/2, Mux112/3
  Mux272/1 -> Mux273/2, Mux193/3
  Mux273/1 -> Mux274/2, Mux234/3
  Mux274/1 -> Mux275/2, Mux255/3
  Mux275/1 -> Mux276/2, Mux266/3
  Mux281/1 -> Mux282/2, Mux122/3
  Mux282/1 -> Mux283/2, Mux203/3
  Mux283/1 -> Mux284/2, Mux244/3
  Mux284/1 -> Mux285/2, Mux265/3
  Mux285/1 -> Mux286/2, Mux276/3
  Mux291/1 -> Mux292/2, Mux132/3
  Mux292/1 -> Mux293/2, Mux213/3
  Mux293/1 -> Mux294/2, Mux254/3
  Mux294/1 -> Mux295/2, Mux275/3
  Mux295/1 -> Mux296/2, Mux286/3
  Mux301/1 -> Mux302/2, Mux142/3
  Mux302/1 -> Mux303/2, Mux223/3
  Mux303/1 -> Mux304/2, Mux264/3
  Mux304/1 -> Mux305/2, Mux285/3
  Mux305/1 -> Mux306/2, Mux296/3
  Mux311/1 -> Mux312/2, Mux152/3
  Mux312/1 -> Mux313/2, Mux233/3
  Mux313/1 -> Mux314/2, Mux274/3
  Mux314/1 -> Mux315/2, Mux295/3
  Mux315/1 -> Mux316/2, Mux306/3
  Mux321/1 -> Mux322/2, Mux162/3
  Mux322/1 -> Mux323/2, Mux243/3
  Mux323/1 -> Mux324/2, Mux284/3
  Mux324/1 -> Mux325/2, Mux305/3
  Mux325/1 -> Mux326/2, Mux316/3
  Mux331/1 -> Mux332/2, Mux172/3
  Mux332/1 -> Mux333/2, Mux253/3
  Mux333/1 -> Mux334/2, Mux294/3
  Mux334/1 -> Mux335/2, Mux315/3
  Mux335/1 -> Mux336/2, Mux326/3
  Mux341/1 -> Mux342/2, Mux182/3
  Mux342/1 -> Mux343/2, Mux263/3
  Mux343/1 -> Mux344/2, Mux304/3
  Mux344/1 -> Mux345/2, Mux325/3
  Mux345/1 -> Mux346/2, Mux336/3
  Mux351/1 -> Mux352/2, Mux192/3
  Mux352/1 -> Mux353/2, Mux273/3
  Mux353/1 -> Mux354/2, Mux314/3
  Mux354/1 -> Mux355/2, Mux335/3
  Mux355/1 -> Mux356/2, Mux346/3
  Mux361/1 -> Mux362/2, Mux202/3
  Mux362/1 -> Mux363/2, Mux283/3
  Mux363/1 -> Mux364/2, Mux324/3
  Mux364/1 -> Mux365/2, Mux345/3
  Mux365/1 -> Mux366/2, Mux356/3
  Mux371/1 -> Mux372/2, Mux212/3
  Mux372/1 -> Mux373/2, Mux293/3
  Mux373/1 -> Mux374/2, Mux334/3
  Mux374/1 -> Mux375/2, Mux355/3
  Mux375/1 -> Mux376/2, Mux366/3
  Mux381/1 -> Mux382/2, Mux222/3
  Mux382/1 -> Mux383/2, Mux303/3
  Mux383/1 -> Mux384/2, Mux344/3
  Mux384/1 -> Mux385/2, Mux365/3
  Mux385/1 -> Mux386/2, Mux376/3
  Mux391/1 -> Mux392/2, Mux232/3
  Mux392/1 -> Mux393/2, Mux313/3
  Mux393/1 -> Mux394/2, Mux354/3
  Mux394/1 -> Mux395/2, Mux375/3
  Mux395/1 -> Mux396/2, Mux386/3
  Mux401/1 -> Mux402/2, Mux242/3
  Mux402/1 -> Mux403/2, Mux323/3
  Mux403/1 -> Mux404/2, Mux364/3
  Mux404/1 -> Mux405/2, Mux385/3
  Mux405/1 -> Mux406/2, Mux396/3
  Mux411/1 -> Mux412/2, Mux252/3
  Mux412/1 -> Mux413/2, Mux333/3
  Mux413/1 -> Mux414/2, Mux374/3
  Mux414/1 -> Mux415/2, Mux395/3
  Mux415/1 -> Mux416/2, Mux406/3
  Mux421/1 -> Mux422/2, Mux262/3
  Mux422/1 -> Mux423/2, Mux343/3
  Mux423/1 -> Mux424/2, Mux384/3
  Mux424/1 -> Mux425/2, Mux405/3
  Mux425/1 -> Mux426/2, Mux416/3
  Mux431/1 -> Mux432/2, Mux272/3
  Mux432/1 -> Mux433/2, Mux353/3
  Mux433/1 -> Mux434/2, Mux394/3
  Mux434/1 -> Mux435/2, Mux415/3
  Mux435/1 -> Mux436/2, Mux426/3
  Mux441/1 -> Mux442/2, Mux282/3
  Mux442/1 -> Mux443/2, Mux363/3
  Mux443/1 -> Mux444/2, Mux404/3
  Mux444/1 -> Mux445/2, Mux425/3
  Mux445/1 -> Mux446/2, Mux436/3
  Mux451/1 -> Mux452/2, Mux292/3
  Mux452/1 -> Mux453/2, Mux373/3
  Mux453/1 -> Mux454/2, Mux414/3
  Mux454/1 -> Mux455/2, Mux435/3
  Mux455/1 -> Mux456/2, Mux446/3
  Mux461/1 -> Mux462/2, Mux302/3
  Mux462/1 -> Mux463/2, Mux383/3
  Mux463/1 -> Mux464/2, Mux424/3
  Mux464/1 -> Mux465/2, Mux445/3
  Mux465/1 -> Mux466/2, Mux456/3
  Mux471/1 -> Mux472/2, Mux312/3
  Mux472/1 -> Mux473/2, Mux393/3
  Mux473/1 -> Mux474/2, Mux434/3
  Mux474/1 -> Mux475/2, Mux455/3
  Mux475/1 -> Mux476/2, Mux466/3
  Mux481/1 -> Mux482/2, Mux322/3
  Mux482/1 -> Mux483/2, Mux403/3
  Mux483/1 -> Mux484/2, Mux444/3
  Mux484/1 -> Mux485/2, Mux465/3
  Mux485/1 -> Mux486/2, Mux476/3
  Mux491/1 -> Mux492/2, Mux332/3
  Mux492/1 -> Mux493/2, Mux413/3
  Mux493/1 -> Mux494/2, Mux454/3
  Mux494/1 -> Mux495/2, Mux475/3
  Mux495/1 -> Mux496/2, Mux486/3
  Mux501/1 -> Mux502/2, Mux342/3
  Mux502/1 -> Mux503/2, Mux423/3
  Mux503/1 -> Mux504/2, Mux464/3
  Mux504/1 -> Mux505/2, Mux485/3
  Mux505/1 -> Mux506/2, Mux496/3
  Mux511/1 -> Mux512/2, Mux352/3
  Mux512/1 -> Mux513/2, Mux433/3
  Mux513/1 -> Mux514/2, Mux474/3
  Mux514/1 -> Mux515/2, Mux495/3
  Mux515/1 -> Mux516/2, Mux506/3
  Mux521/1 -> Mux522/2, Mux362/3
  Mux522/1 -> Mux523/2, Mux443/3
  Mux523/1 -> Mux524/2, Mux484/3
  Mux524/1 -> Mux525/2, Mux505/3
  Mux525/1 -> Mux526/2, Mux516/3
  Mux531/1 -> Mux532/2, Mux372/3
  Mux532/1 -> Mux533/2, Mux453/3
  Mux533/1 -> Mux534/2, Mux494/3
  Mux534/1 -> Mux535/2, Mux515/3
  Mux535/1 -> Mux536/2, Mux526/3
  Mux541/1 -> Mux542/2, Mux382/3
  Mux542/1 -> Mux543/2, Mux463/3
  Mux543/1 -> Mux544/2, Mux504/3
  Mux544/1 -> Mux545/2, Mux525/3
  Mux545/1 -> Mux546/2, Mux536/3
  Mux551/1 -> Mux552/2, Mux392/3
  Mux552/1 -> Mux553/2, Mux473/3
  Mux553/1 -> Mux554/2, Mux514/3
  Mux554/1 -> Mux555/2, Mux535/3
  Mux555/1 -> Mux556/2, Mux546/3
  Mux561/1 -> Mux562/2, Mux402/3
  Mux562/1 -> Mux563/2, Mux483/3
  Mux563/1 -> Mux564/2, Mux524/3
  Mux564/1 -> Mux565/2, Mux545/3
  Mux565/1 -> Mux566/2, Mux556/3
  Mux571/1 -> Mux572/2, Mux412/3
  Mux572/1 -> Mux573/2, Mux493/3
  Mux573/1 -> Mux574/2, Mux534/3
  Mux574/1 -> Mux575/2, Mux555/3
  Mux575/1 -> Mux576/2, Mux566/3
  Mux581/1 -> Mux582/2, Mux422/3
  Mux582/1 -> Mux583/2, Mux503/3
  Mux583/1 -> Mux584/2, Mux544/3
  Mux584/1 -> Mux585/2, Mux565/3
  Mux585/1 -> Mux586/2, Mux576/3
  Mux591/1 -> Mux592/2, Mux432/3
  Mux592/1 -> Mux593/2, Mux513/3
  Mux593/1 -> Mux594/2, Mux554/3
  Mux594/1 -> Mux595/2, Mux575/3
  Mux595/1 -> Mux596/2, Mux586/3
  Mux601/1 -> Mux602/2, Mux442/3
  Mux602/1 -> Mux603/2, Mux523/3
  Mux603/1 -> Mux604/2, Mux564/3
  Mux604/1 -> Mux605/2, Mux585/3
  Mux605/1 -> Mux606/2, Mux596/3
  Mux611/1 -> Mux612/2, Mux452/3
  Mux612/1 -> Mux613/2, Mux533/3
  Mux613/1 -> Mux614/2, Mux574/3
  Mux614/1 -> Mux615/2, Mux595/3
  Mux615/1 -> Mux616/2, Mux606/3
  Mux621/1 -> Mux622/2, Mux462/3
  Mux622/1 -> Mux623/2, Mux543/3
  Mux623/1 -> Mux624/2, Mux584/3
  Mux624/1 -> Mux625/2, Mux605/3
  Mux625/1 -> Mux626/2, Mux616/3
  Mux631/1 -> Mux632/2, Mux472/3
  Mux632/1 -> Mux633/2, Mux553/3
  Mux633/1 -> Mux634/2, Mux594/3
  Mux634/1 -> Mux635/2, Mux615/3
  Mux635/1 -> Mux636/2, Mux626/3
  Mux641/1 -> Mux642/2, Mux482/3
  Mux642/1 -> Mux643/2, Mux563/3
  Mux643/1 -> Mux644/2, Mux604/3
  Mux644/1 -> Mux645/2, Mux625/3
  Mux645/1 -> Mux646/2, Mux636/3

== system c960x4096_x14_7_r2013b_frb/vacc/vacc/yy/bit_sel3/bus_create ==
  in1 : Inport
  in2 : Inport  Port=2
  in3 : Inport  Port=3
  in4 : Inport  Port=4
  in5 : Inport  Port=5
  in6 : Inport  Port=6
  in7 : Inport  Port=7
  in8 : Inport  Port=8
  concatenate : xbsIndex_r4/Concat  num_inputs=8  dbl_ovrd=off  block_type=concat
  reinterpret{1..8} (8 alike) : xbsIndex_r4/Reinterpret  force_arith_type=on  arith_type=Unsigned  force_bin_pt=on  bin_pt=0  block_type=reinterpret
  bus_out : Outport
  wires:
  concatenate/1 -> bus_out/1
  in1/1 -> reinterpret1/1
  reinterpret1/1 -> concatenate/1
  in2/1 -> reinterpret2/1
  reinterpret2/1 -> concatenate/2
  in3/1 -> reinterpret3/1
  reinterpret3/1 -> concatenate/3
  in4/1 -> reinterpret4/1
  reinterpret4/1 -> concatenate/4
  in5/1 -> reinterpret5/1
  reinterpret5/1 -> concatenate/5
  in6/1 -> reinterpret6/1
  reinterpret6/1 -> concatenate/6
  in7/1 -> reinterpret7/1
  reinterpret7/1 -> concatenate/7
  in8/1 -> reinterpret8/1
  reinterpret8/1 -> concatenate/8
